simulink model "Prac_2_Q3_2"  (R2020a)
settings: Solver=FixedStepAuto  StartTime=0  StopTime=21600  FixedStep=3  RelTol=1e-3
values from neighbouring files (symbols this model uses):
  Cr = 100000    [Prac_2.m]
  K = 100    [Prac_2.m]
  Qf = 1000    [Prac_2.m]
  Qr2 = 2500    [Prac_2.m]
  T0 = 5    [Prac_2.m]
  Ta = 0    [Prac_2.m]
  Toff = 26    [Prac_2.m]
  Ton = 24    [Prac_2.m]
settings Model: Creator=mluser  LastModifiedBy=kaibr
settings DebuggingCC: SFMachineParentedDataDiag=error

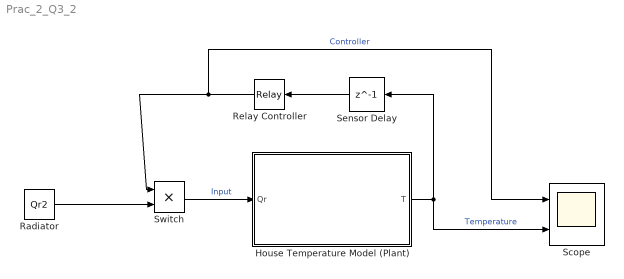
== system Prac_2_Q3_2 ==
  House Temperature Model (Plant) : Subsystem
  Radiator : Constant  Value=Qr2
  Relay Controller : Relay  OnSwitchValue=Toff  OffSwitchValue=Ton  OnOutputValue=0  OffOutputValue=1
  Scope : Scope  NumInputPorts=2
  Sensor Delay : Delay  DelayLength=1  InitialCondition=0
  Switch : Product
  wires:
  Radiator/1 -> Switch/2
  House Temperature Model (Plant)/1(T) -> Scope/2, Sensor Delay/1  "Temperature"
  Switch/1 -> House Temperature Model (Plant)/1(Qr)  "Input"
  Sensor Delay/1 -> Relay Controller/1
  Relay Controller/1 -> Scope/1, Switch/1  "Controller"

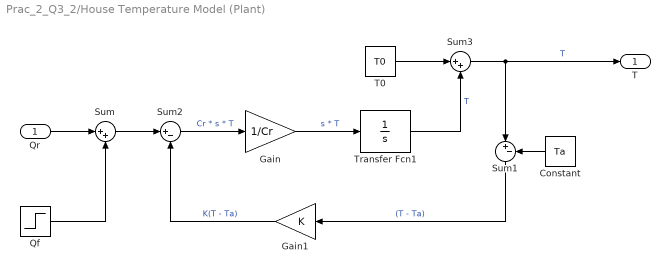
== system Prac_2_Q3_2/House Temperature Model (Plant) ==
  Qr : Inport
  Constant : Constant  Value=Ta
  Gain : Gain  Gain=1/Cr
  Gain1 : Gain  Gain=K
  Qf : Step  Time=7200  After=Qf  SampleTime=0
  Sum : Sum  Inputs=|++
  Sum1 : Sum  Inputs=|+-
  Sum2 : Sum  Inputs=|+-
  Sum3 : Sum  Inputs=|++
  T0 : Constant  Value=T0
  Transfer Fcn1 : TransferFcn  Denominator=[1 0]
  T : Outport
  wires:
  Sum3/1 -> T/1, Sum1/1  "T"
  T0/1 -> Sum3/1
  Transfer Fcn1/1 -> Sum3/2  "T"
  Qf/1 -> Sum/2
  Sum2/1 -> Gain/1  "Cr * s * T"
  Sum1/1 -> Gain1/1  "(T - Ta)"
  Gain/1 -> Transfer Fcn1/1  "s * T"
  Constant/1 -> Sum1/2
  Sum/1 -> Sum2/1
  Gain1/1 -> Sum2/2  "K(T - Ta)"
  Qr/1 -> Sum/1
